simulink model "WindTurbineNM80"  (R2025b)
settings: Solver=VariableStepAuto  StartTime=0.0  StopTime=1000.0  MaxStep=0.02  RelTol=1e-3  AbsTol=1e-3  EnableMultiTasking=on
InitFcn:
  | WindTurbineNM80_init
values from neighbouring files (symbols this model uses):
  Ki = 0.5    [WindTurbineNM80_init.m]
  Kp = -[1.50 1.10 0.95 0.75 0.60 0.40 0.30 0.25]    [WindTurbineNM80_init.m]
  Lomg = 0:0.1:2*omgn    [WindTurbineNM80_init.m]
  Ltorque = zeros(1, length(Lomg))    [WindTurbineNM80_init.m]
  P0 = block.DialogPrm(1).Data    [Sbem.m]    (also in V10_init.mat = [0.0256690203 0 0.1920105638 0 1.7253273454 0.0016163595 0 0; V12_init.mat = [0.0307356949 0 0.2300256376 0 1.7632116641 0.0024078403 0 0; V15_init.mat = [0.0285896181 0 0.2236008103 0 1.8055130146 0.0031083935 0 5; V20_init.mat = [0.0174352214 0 0.1599644548 0 1.8055130193 0.0031083935 0 1)
  P1 = [rho, kp]    [NM80.m]    (also in NM92.m; Sbem.m = block.DialogPrm(2).Data)
  P2 = [R Nb Jb kb mt dt kt nu Jr dr kr Jg Un Pn omgn If p]    [NM80.m]    (also in NM92.m; Sbem.m = block.DialogPrm(3).Data)
  P3 = [r; c; thetat; th]    [NM80.m]    (also in NM92.m = [r; c; thetat]; Sbem.m = block.DialogPrm(4).Data)
  P4 = [Vn, lambdan, thetan]    [NM80.m]    (also in NM92.m)
  Pc = [omgA omgB omgC omgD omgE MB MC ME Kopt]    [WindTurbineNM80_init.m]
  Ptheta = [0 1 2 5 10 15 20 30]    [WindTurbineNM80_init.m]
  theta0 = 0.1    [V10_init.mat]    (also in V12_init.mat; V15_init.mat = 5.6378340943; V20_init.mat = 15.771114223; V25_init.mat = 22.7706169843)
  V0 = 10    [V10_init.mat]    (also in V12_init.mat = 12; V15_init.mat = 15; V20_init.mat = 20; V25_init.mat = 25)
libraries: sim3dlib x2, simulink x1
settings Model: Creator=ihoutzager  LastModifiedBy=ihout
settings SolverCC: AutoScaleAbsTol=off  AlgebraicLoopSolver=TrustRegion
settings DataIOCC: LimitDataPoints=on  SaveFormat=Array  SignalLoggingSaveFormat=ModelDataLogs  SaveOutput=off  SignalLogging=off  SaveTime=off  ReturnWorkspaceOutputs=off  SignalLoggingName=sigsOut
settings OptimizationCC: InitFltsAndDblsToZero=on  LifeSpan=inf
settings DebuggingCC: AlgebraicLoopMsg=none  SaveWithParameterizedLinksMsg=none  UnderspecifiedInitializationDetection=Classic  MergeDetectMultiDrivingBlocksExec=none  SignalResolutionControl=TryResolveAllWithWarning  MultiTaskDSMMsg=warning  MultiTaskCondExecSysMsg=none  FcnCallInpInsideContextMsg=warning  UnconnectedInputMsg=warning  UnconnectedOutputMsg=warning  UnconnectedLineMsg=warning  SFUnexpectedBacktrackingDiag=warning  SFNoUnconditionalDefaultTransitionDiag=warning  SFExecutionAtInitializationDiag=none  ArithmeticOperatorsInVariantConditions=warning
settings HardwareCC: ProdBitPerPointer=32.0  ProdBitPerSizeT=32.0  ProdBitPerPtrDiffT=32.0  ProdLargestAtomicFloat=None  ProdIntDivRoundTo=Undefined  ProdEndianess=Unspecified  ProdWordSize=32.0  ProdHWDeviceType=32-bit Generic  TargetUnknown=on
settings ModelReferenceCC: PropagateSignalLabelsOutOfModel=off
settings SFSimCC: SimParseCustomCode=off
settings RTWCC: GPUComputeCapability=3.5
settings CodeAppCC: StateflowObjectComments=on
settings GRTTargetCC: TargetFcnLib=ansi_tfl_tmw.mat  TargetLangStandard=C89/C90 (ANSI)  CombineOutputUpdateFcns=off  GRTInterface=on
settings ConfigComp: CovMetricSettings=dw  CovSaveCumulativeToWorkspaceVar=on  CovSaveSingleToWorkspaceVar=on

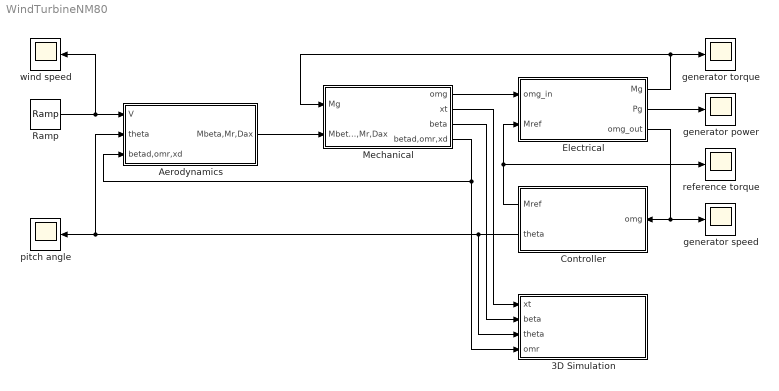
== system WindTurbineNM80 ==
  3D Simulation : Subsystem
  Aerodynamics : Subsystem
  Controller : Subsystem
  Electrical : Subsystem
  Mechanical : Subsystem
  Ramp : simulink/Sources/Ramp  slope=0.02  start=100  InitialOutput=V0
  generator power : Scope
      settings: TimeSpan=29.23076923076923  ActiveDisplayYMinimum=1.8990232335376493E+6  ActiveDisplayYMaximum=8.8179371513424478E+6  DataLoggingVariableName=ScopeData3
  generator speed : Scope
      settings: ActiveDisplayYMinimum=62.485741146490142  ActiveDisplayYMaximum=70.982692485822966  DataLoggingVariableName=ScopeData4
  generator torque : Scope
      settings: ActiveDisplayYMinimum=-2749.5211903948921  ActiveDisplayYMaximum=24745.690713554031
  pitch angle : Scope
      settings: ActiveDisplayYMinimum=16.304990778596967  ActiveDisplayYMaximum=20.832866708682104  DataLoggingVariableName=ScopeData2
  reference torque : Scope
      settings: ActiveDisplayYMinimum=2000  ActiveDisplayYMaximum=13000  DataLoggingVariableName=ScopeData5
  wind speed : Scope
      settings: ActiveDisplayYMinimum=3.5895500000000005  ActiveDisplayYMaximum=17.69405
  wires:
  Electrical/1(Mg) -> Mechanical/1(Mg), generator torque/1
  Mechanical/1(omg) -> Electrical/1(omg_in)
  Mechanical/4(betad,omr,xd) -> Aerodynamics/3(betad,omr,xd), 3D Simulation/4(omr)
  Controller/1(Mref) -> reference torque/1, Electrical/2(Mref)
  Electrical/3(omg_out) -> Controller/1(omg), generator speed/1
  Controller/2(theta) -> pitch angle/1, Aerodynamics/2(theta), 3D Simulation/3(theta)
  Aerodynamics/1(Mbeta,Mr,Dax) -> Mechanical/2(Mbeta,Mr,Dax)
  Ramp/1 -> wind speed/1, Aerodynamics/1(V)
  Electrical/2(Pg) -> generator power/1
  Mechanical/2(xt) -> 3D Simulation/1(xt)
  Mechanical/3(beta) -> 3D Simulation/2(beta)

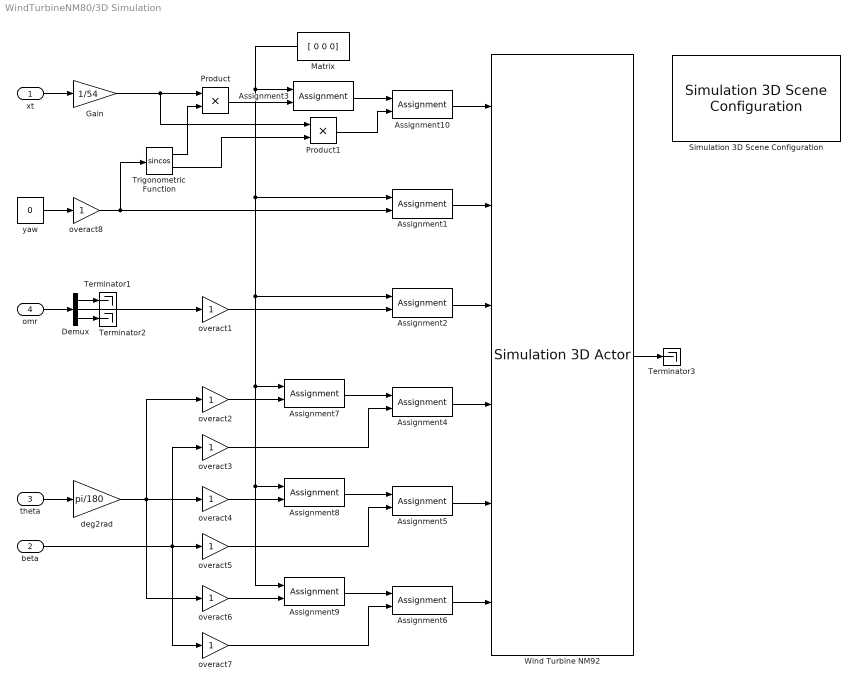
== system WindTurbineNM80/3D Simulation ==
  xt : Inport
  beta : Inport  Port=2
  theta : Inport  Port=3
  omr : Inport  Port=4
  Assignment{1,7..9} (4 alike) : Assignment  DiagnosticForDimensions=Warning  IndexOptions=Index vector (dialog)  Indices=3  OutputSizes=1
  Assignment10 : Assignment  DiagnosticForDimensions=Warning  IndexOptions=Index vector (dialog)  Indices=2  OutputSizes=1
  Assignment2 : Assignment  DiagnosticForDimensions=Warning  IndexOptions=Index vector (dialog)  Indices=2  OutputSizes=1
  Assignment{3..6} (4 alike) : Assignment  DiagnosticForDimensions=Warning  IndexOptions=Index vector (dialog)  Indices=1  OutputSizes=1
  Demux : Demux  Outputs=3
  Gain : Gain  Gain=1/54
  Matrix : Constant  Value=[ 0 0 0]  VectorParams1D=off
  Product : Product
  Product1 : Product
  Simulation 3D Scene Configuration : sim3dlib/Simulation 3D Scene Configuration  Priority=0  ProjectFormat=Default Scenes  SceneDesc=Empty scene  ProjectName=C:\Program Files\MATLAB\R2025b\toolbox\shared\sim3d_projects\automotive_project_windows\UE\WindowsNoEditor\VehicleSimulation.exe  ScenePath=/Game/Maps/HwStrght  EnableOpenDRIVE=off  vehTagList={'Custom';'Front';'Quadcopter';'Scene Origin';'WindTurbineNM92'}  vehTag=Front  AttachedCameraRelativeTranslation=[0 0 0]  FreeCameraDefaultInitialTranslation=[-6, 0, 2]  AttachedCameraRelativeRotation=[0 0 0]  FreeCameraDefaultInitialRotation=[0, -15, 0]  ViewpointName=Front  FreeCameraInitialTranslation=[0 120 60]  ViewpointTranslation=[0 0 0]  FreeCameraInitialRotation=[0 0 -90]  ViewpointRotation=[0 0 0]  OpVisEn=off  Ts=.02  EnableWindow=on  EnableRemoteAccess=off  EnableWeather=off  SunAzimuth=90  SunAltitude=40.0  EnableGeospatialSun=off  Latitude=0  Longitude=0  Date=2023-01-01  Time=10:30:00  GeoTimeZone=-5.0  SunDaylightSaving=off  wind=1  clouds=10  EnableVolumetricClouds=off  CloudCoverage=0  CloudAltitude=6  fog=0  rain=0  RaindropsEffect=off  SnowDensity=0  EnableGeospatial=off  TilesetSource=Earth terrain  UseTrueOrigin=off  OriginHeight=200  OriginLatitude=40.744652  OriginLongitude=-73.988864  MapStyle=Aerial  AdditionalAssetIDs=[]  UseAdvancedSunSky=off  SolarTime=11  TimeZone=-5  Day=21  Month=9  Year=2022  UseDaylightSavingTime=on  DSTStartDay=10  DSTStartMonth=3  DSTEndDay=3  DSTEndMonth=11  DSTSwitchHour=2  sensorTag=MainCamera1  sensorId=1  sensorName=MainCamera1  mountLoc=Origin  offsetFlag=off  tmountOffset=[0, 0, 0]  rmountOffset=[0, 0, 0]  HorizontalResolution=1280  VerticalResolution=720  HorizontalFOV=60  mountPoint=[0 0 0]  mountOrientation=[0 0 0]  aMode=5  ID=1  GeoTrigger=Inactive  ViewNameList={'Custom', 'Front'}  ViewTranslationList={'[0 0 0]', '[0 120 60]'}  ViewRotationList={'[0 0 0]', '[0 0 -90]'}
      settings: LibrarySourceBlock=sl3dlib/Simulation 3D/Simulation 3D Scene Configuration
  Terminator1 : Terminator
  Terminator2 : Terminator
  Terminator3 : Terminator
  Trigonometric Function : Trigonometry  Operator=sincos
  Wind Turbine NM92 : sim3dlib/Simulation 3D Actor  Priority=1  ActorName=WindTurbineNM92  ParentName=Front  Operation=Create at setup  InitScriptText=|  SampleTime=-1  Translation=[0 0 0]  Rotation=[0 0 0]  Scale=[1 1 1]  InputsText=|  aMode=5  ActorTag=WindTurbineNM92  ActorType=Sim3dActor  ID=C
      InitScriptText=|
      | NM92.FoundationPile = sim3d.Actor(ActorName='FoundationPile',...
      |     Translation=[0 0 0],...
      |     Mobility=sim3d.utils.MobilityTypes.Static);
      | add(World,NM92.FoundationPile,Actor);
      | load(NM92.FoundationPile,'actors3d\NM92_FoundationPile.x3d')
      | 
      | NM92.DeckSupportPlate1 = sim3d.Actor(ActorName='DeckSupportPlate1',...
      |     Mobility=sim3d.utils.MobilityTypes.Static);
      | add(World,NM92.DeckSupportPlate1,Actor);
      | load(NM92.DeckSupportPlate1,'actors3d\NM92_DeckSupportPlate1.x3d')
      | 
      | NM92.DeckSupportPlate2 = sim3d.Actor(ActorName='DeckSupportPlate2',...
      |     Mobility=sim3d.utils.MobilityTypes.Static);
      | add(World,NM92.DeckSupportPlate2,Actor);
      | load(NM92.DeckSupportPlate2,'actors3d\NM92_DeckSupportPlate2.x3d')
      | 
      | NM92.DeckSupport1 = sim3d.Actor(ActorName='DeckSupport1',...
      |     Mobility=sim3d.utils.MobilityTypes.Static);
      | add(World,NM92.DeckSupport1,Actor);
      | load(NM92.DeckSupport1,'actors3d\NM92_DeckSupport1.x3d')
      | 
      | NM92.DeckSupport2 = sim3d.Actor(ActorName='DeckSupport2',...
      |     Mobility=sim3d.utils.MobilityTypes.Static);
      | add(World,NM92.DeckSupport2,Actor);
      | load(NM92.DeckSupport2,'actors3d\NM92_DeckSupport2.x3d')
      | 
      | NM92.Deck = sim3d.Actor(ActorName='Deck',...
      |     Mobility=sim3d.utils.MobilityTypes.Static);
      | add(World,NM92.Deck,Actor);
      | load(NM92.Deck,'actors3d\NM92_Deck.x3d')
      | 
      | NM92.DeckRailing = sim3d.Actor(ActorName='DeckRailing',...
      |     Mobility=sim3d.utils.MobilityTypes.Static);
      | add(World,NM92.DeckRailing,Actor);
      | load(NM92.DeckRailing,'actors3d\NM92_DeckRailing.x3d')
      | 
      | NM92.ForeAftJoint = sim3d.Actor(ActorName='ForeAftJoint',...
      |     Translation=[0 0 14],...
      |     Mobility=sim3d.utils.MobilityTypes.Movable);
      | add(World,NM92.ForeAftJoint,NM92.FoundationPile)
      | 
      | NM92.Tower = sim3d.Actor(ActorName='Tower',...
      |     Translation=[0 0 -14],...
      |     Mobility=sim3d.utils.MobilityTypes.Movable);
      | add(World,NM92.Tower,NM92.ForeAftJoint);
      | load(NM92.Tower,'actors3d\NM92_Tower.x3d')
      | 
      | NM92.Door = sim3d.Actor(ActorName='Door',...
      |     Translation=[0 0 -14],...
      |     Mobility=sim3d.utils.MobilityTypes.Movable);
      | add(World,NM92.Door,NM92.ForeAftJoint);
      | load(NM92.Door,'actors3d\NM92_Door.x3d')
      | 
      | NM92.YawJoint = sim3d.Actor(ActorName='YawJoint',...
      |     Translation=[0 0 68],...
      |     Mobility=sim3d.utils.MobilityTypes.Movable);
      | add(World,NM92.YawJoint,NM92.Tower)
      | 
      | NM92.NacelleSpoiler = sim3d.Actor(ActorName='NacelleSpoiler',...
      |     Translation=[0 0 -68],...
      |     Mobility=sim3d.utils.MobilityTypes.Movable);
      | add(World,NM92.NacelleSpoiler,NM92.YawJoint);
      | load(NM92.NacelleSpoiler,'actors3d\NM92_NacelleSpoiler.x3d')
      | 
      | NM92.NacelleSpoilerMesh = sim3d.Actor(ActorName='NacelleSpoilerMesh',...
      |     Mobility=sim3d.utils.MobilityTypes.Movable);
      | add(World,NM92.NacelleSpoilerMesh,NM92.NacelleSpoiler);
      | load(NM92.NacelleSpoilerMesh,'actors3d\NM92_NacelleSpoilerMesh.x3d')
      | 
      | NM92.NacelleSides = sim3d.Actor(ActorName='NacelleSides',...
      |     Mobility=sim3d.utils.MobilityTypes.Movable);
      | add(world,NM92.NacelleSides,NM92.NacelleSpoiler);
      | load(NM92.NacelleSides,'actors3d\NM92_NacelleSides.x3d')
      | 
      | NM92.HubConnect = sim3d.Actor(ActorName='HubConnect',...
      |     Mobility=sim3d.utils.MobilityTypes.Movable);
      | add(World,NM92.HubConnect,NM92.NacelleSpoiler);
      | load(NM92.HubConnect,'actors3d\NM92_HubConnect.x3d')
      | 
      | NM92.RotationAxis = sim3d.Actor(ActorName='RotationAxis',...
      |     Translation=[-0.039169 2.146902 69.95571],...
      |     Rotation=[-0.0698124 0 0],...
      |     Mobility=sim3d.utils.MobilityTypes.Movable);
      | add(World,NM92.RotationAxis,NM92.HubConnect)
      | 
      | NM92.RotationJoint = sim3d.Actor(ActorName='RotationJoint',...
      |     Mobility=sim3d.utils.MobilityTypes.Movable);
      | add(World,NM92.RotationJoint,NM92.RotationAxis)
      | 
      | NM92.RotationInverse = sim3d.Actor(ActorName='RotationInverse',...
      |     Rotation=[0.0698124 0 0],...
      |     Mobility=sim3d.utils.MobilityTypes.Movable);
      | add(World,NM92.RotationInverse,NM92.RotationJoint)
      | 
      | NM92.Hub = sim3d.Actor(ActorName='Hub',...
      |     Translation=[0.039169 -2.146902 -69.95571],...
      |     Mobility=sim3d.utils.MobilityTypes.Movable);
      | add(World,NM92.Hub,NM92.RotationInverse);
      | load(NM92.Hub,'actors3d\NM92_Hub.x3d')
      |  
      | NM92.HubHatch1 = sim3d.Actor(ActorName='HubHatch1',...
      |     Mobility=sim3d.utils.MobilityTypes.Movable);
      | add(World,NM92.HubHatch1,NM92.Hub);
      | load(NM92.HubHatch1,'actors3d\NM92_HubHatch1.x3d')
      | 
      | NM92.HubHatch2 = sim3d.Actor(ActorName='HubHatch2',...
      |     Mobility=sim3d.utils.MobilityTypes.Movable);
      | add(World,NM92.HubHatch2,NM92.Hub);
      | load(NM92.HubHatch2,'actors3d\NM92_HubHatch2.x3d')
      | 
      | NM92.HubHatch3 = sim3d.Actor(ActorName='HubHatch3',...
      |     Mobility=sim3d.utils.MobilityTypes.Movable);
      | add(World,NM92.HubHatch3,NM92.Hub);
      | load(NM92.HubHatch3,'actors3d\NM92_HubHatch3.x3d')
      | 
      | NM92.RotorAxis = sim3d.Actor(ActorName='RotorAxis',...
      |     Translation=[-0.035752 3.576152 70.059258],...
      |     Rotation=[-0.0698124 0 0],...
      |     Mobility=sim3d.utils.MobilityTypes.Movable);
      | add(World,NM92.RotorAxis,NM92.Hub)
      | 
      | NM92.BladeAxis1= sim3d.Actor(ActorName='BladeAxis1',...
      |     Rotation=[0 -pi*2/3 0],...
      |     Mobility=sim3d.utils.MobilityTypes.Movable);
      | add(World,NM92.BladeAxis1,NM92.RotorAxis)
      | 
      | NM92.BladeJoint1= sim3d.Actor(ActorName='BladeJoint1',...
      |     Mobility=sim3d.utils.MobilityTypes.Movable);
      | add(World,NM92.BladeJoint1,NM92.BladeAxis1)
      | 
      | NM92.BladeInverse1 = sim3d.Actor(ActorName='BladeInverse1',...
      |     Rotation=[0.0698124 pi*2/3 pi],...
      |     Mobility=sim3d.utils.MobilityTypes.Movable);
      | add(World,NM92.BladeInverse1,NM92.BladeJoint1)
      | 
      | NM92.Blade1 = sim3d.Actor(ActorName='Blade1',...
      |     Translation=[0.035752 -3.576152 -70.059258],...
      |     Mobility=sim3d.utils.MobilityTypes.Movable);
      | add(World,NM92.Blade1,NM92.BladeInverse1);
      | load(NM92.Blade1,'actors3d\NM92_Blade1.x3d')
      | 
      | NM92.BladeAxis2= sim3d.Actor(ActorName='BladeAxis2',...
      |     Rotation=[0 pi*2/3 0],...
      |     Mobility=sim3d.utils.MobilityTypes.Movable);
      | add(World,NM92.BladeAxis2,NM92.RotorAxis)
      | 
      | NM92.BladeJoint2= sim3d.Actor(ActorName='BladeJoint2',...
      |     Mobility=sim3d.utils.MobilityTypes.Movable);
      | add(World,NM92.BladeJoint2,NM92.BladeAxis2)
      | 
      | NM92.BladeInverse2 = sim3d.Actor(ActorName='BladeInverse2',...
      |     Rotation=[0.0698124 -pi*2/3 pi],...
      |     Mobility=sim3d.utils.MobilityTypes.Movable);
      | add(World,NM92.BladeInverse2,NM92.BladeJoint2)
      | 
      | NM92.Blade2 = sim3d.Actor(ActorName='Blade2',...
      |     Translation=[0.035752 -3.576152 -70.059258],...
      |     Mobility=sim3d.utils.MobilityTypes.Movable);
      | add(World,NM92.Blade2,NM92.BladeInverse2);
      | load(NM92.Blade2,'actors3d\NM92_Blade2.x3d')
      | 
      | NM92.BladeAxis3= sim3d.Actor(ActorName='BladeAxis3',...
      |     Rotation=[0 0 0],...
      |     Mobility=sim3d.utils.MobilityTypes.Movable);
      | add(World,NM92.BladeAxis3,NM92.RotorAxis)
      | 
      | NM92.BladeJoint3= sim3d.Actor(ActorName='BladeJoint3',...
      |     Mobility=sim3d.utils.MobilityTypes.Movable);
      | add(World,NM92.BladeJoint3,NM92.BladeAxis3)
      | 
      | NM92.BladeInverse3 = sim3d.Actor(ActorName='BladeInverse3',...
      |     Rotation=[0.0698124 0 pi],...
      |     Mobility=sim3d.utils.MobilityTypes.Movable);
      | add(World,NM92.BladeInverse3,NM92.BladeJoint3)
      | 
      | NM92.Blade3 = sim3d.Actor(ActorName='Blade3',...
      |     Translation=[0.035752 -3.576152 -70.059258],...
      |     Mobility=sim3d.utils.MobilityTypes.Movable);
      | add(World,NM92.Blade3,NM92.BladeInverse3);
      | load(NM92.Blade3,'actors3d\NM92_Blade3.x3d')
      InputsText=|
      | ForeAftJoint.Rotation        
      | YawJoint.Rotation           
      | RotationJoint.AngularVelocity
      | BladeJoint1.Rotation         
      | BladeJoint2.Rotation         
      | BladeJoint3.Rotation
  deg2rad : Gain  Gain=pi/180
  overact{1..8} (8 alike) : Gain
  yaw : Constant  Value=0
  wires:
  Gain/1 -> Product/1, Product1/1
  Demux/2 -> overact1/1
  omr/1 -> Demux/1
  deg2rad/1 -> overact6/1, overact2/1, overact4/1
  Demux/1 -> Terminator1/1
  Demux/3 -> Terminator2/1
  Wind Turbine NM92/1 -> Terminator3/1
  Matrix/1 -> Assignment1/1, Assignment2/1, Assignment9/1, Assignment8/1, Assignment7/1, Assignment3/1
  Assignment1/1 -> Wind Turbine NM92/2
  yaw/1 -> overact8/1
  overact8/1 -> Trigonometric Function/1, Assignment1/2
  overact1/1 -> Assignment2/2
  Assignment7/1 -> Assignment4/1
  Assignment8/1 -> Assignment5/1
  Assignment9/1 -> Assignment6/1
  overact3/1 -> Assignment4/2
  overact2/1 -> Assignment7/2
  overact5/1 -> Assignment5/2
  overact7/1 -> Assignment6/2
  overact4/1 -> Assignment8/2
  overact6/1 -> Assignment9/2
  xt/1 -> Gain/1
  Assignment2/1 -> Wind Turbine NM92/3
  Assignment4/1 -> Wind Turbine NM92/4
  Assignment5/1 -> Wind Turbine NM92/5
  Assignment6/1 -> Wind Turbine NM92/6
  Assignment10/1 -> Wind Turbine NM92/1
  Assignment3/1 -> Assignment10/1
  Product/1 -> Assignment3/2
  Trigonometric Function/2 -> Product1/2
  Trigonometric Function/1 -> Product/2
  Product1/1 -> Assignment10/2
  beta/1 -> overact7/1, overact3/1, overact5/1
  theta/1 -> deg2rad/1

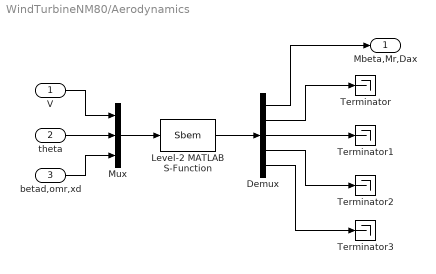
== system WindTurbineNM80/Aerodynamics ==
  V : Inport
  theta : Inport  Port=2
  betad,omr,xd : Inport  Port=3
  Demux : Demux  Outputs=[3,1,1,1,1]
      settings: DisplayOption=none
  Level-2 MATLAB S-Function : M-S-Function  FunctionName=Sbem  Parameters=P0,P1,P2,P3,P4
  Mux : Mux  Inputs=3
  Terminator{,1..3} (4 alike) : Terminator
  Mbeta,Mr,Dax : Outport
  wires:
  theta/1 -> Mux/2
  V/1 -> Mux/1
  betad,omr,xd/1 -> Mux/3
  Mux/1 -> Level-2 MATLAB S-Function/1
  Level-2 MATLAB S-Function/1 -> Demux/1
  Demux/1 -> Mbeta,Mr,Dax/1
  Demux/3 -> Terminator1/1
  Demux/4 -> Terminator2/1
  Demux/5 -> Terminator3/1
  Demux/2 -> Terminator/1

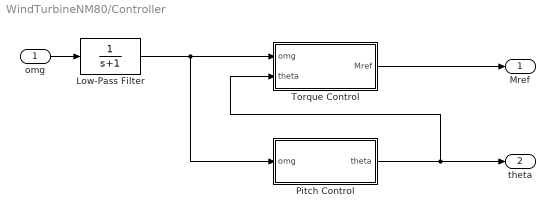
== system WindTurbineNM80/Controller ==
  omg : Inport
  Low-Pass Filter : TransferFcn  Denominator=[1 1]
  Pitch Control : Subsystem
  Torque Control : Subsystem
  Mref : Outport
  theta : Outport  Port=2
  wires:
  omg/1 -> Low-Pass Filter/1
  Low-Pass Filter/1 -> Pitch Control/1(omg), Torque Control/1(omg)
  Pitch Control/1(theta) -> Torque Control/2(theta), theta/1
  Torque Control/1(Mref) -> Mref/1

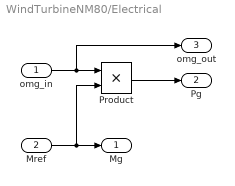
== system WindTurbineNM80/Electrical ==
  omg_in : Inport
  Mref : Inport  Port=2
  Product : Product  RndMeth=Zero
  Mg : Outport
  Pg : Outport  Port=2
  omg_out : Outport  Port=3
  wires:
  Product/1 -> Pg/1
  omg_in/1 -> Product/1, omg_out/1
  Mref/1 -> Mg/1, Product/2

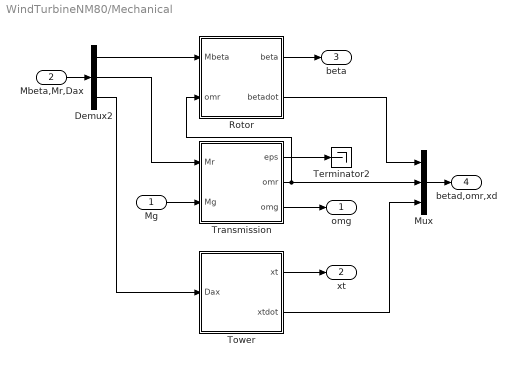
== system WindTurbineNM80/Mechanical ==
  Mg : Inport
  Mbeta,Mr,Dax : Inport  Port=2
  Demux2 : Demux  Outputs=3
      settings: DisplayOption=none
  Mux : Mux  Inputs=3
  Rotor : Subsystem
  Terminator2 : Terminator
  Tower : Subsystem
  Transmission : Subsystem
  omg : Outport
  xt : Outport  Port=2
  beta : Outport  Port=3
  betad,omr,xd : Outport  Port=4
  wires:
  Transmission/3(omg) -> omg/1
  Rotor/2(betadot) -> Mux/1
  Transmission/2(omr) -> Mux/2, Rotor/2(omr)
  Mux/1 -> betad,omr,xd/1
  Transmission/1(eps) -> Terminator2/1
  Tower/2(xtdot) -> Mux/3
  Tower/1(xt) -> xt/1
  Mbeta,Mr,Dax/1 -> Demux2/1
  Mg/1 -> Transmission/2(Mg)
  Demux2/1 -> Rotor/1(Mbeta)
  Demux2/3 -> Tower/1(Dax)
  Demux2/2 -> Transmission/1(Mr)
  Rotor/1(beta) -> beta/1

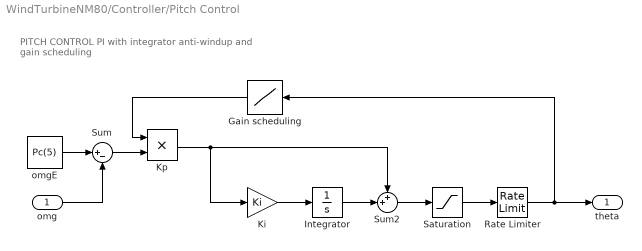
== system WindTurbineNM80/Controller/Pitch Control ==
  note: PITCH CONTROL
      | PI with integrator anti-windup and gain scheduling
  omg : Inport
  Gain scheduling : Lookup  InputValues=Ptheta  Table=Kp  LookUpMeth=Interpolation-Use End Values  SaturateOnIntegerOverflow=off
  Integrator : Integrator  InitialCondition=theta0  LimitOutput=on  UpperSaturationLimit=90  LowerSaturationLimit=P4(3)
  Ki : Gain  Gain=Ki
  Kp : Product  RndMeth=Zero
  Rate Limiter : RateLimiter  RisingSlewLimit=4  FallingSlewLimit=-4  SampleTimeMode=inherited
  Saturation : Saturate  UpperLimit=90  LowerLimit=P4(3)
  Sum : Sum  Inputs=|+-
  Sum2 : Sum  Inputs=++|
  omgE : Constant  Value=Pc(5)
  theta : Outport
  wires:
  omgE/1 -> Sum/1
  Sum/1 -> Kp/2
  Integrator/1 -> Sum2/2
  Sum2/1 -> Saturation/1
  Ki/1 -> Integrator/1
  Kp/1 -> Sum2/1, Ki/1
  omg/1 -> Sum/2
  Gain scheduling/1 -> Kp/1
  Saturation/1 -> Rate Limiter/1
  Rate Limiter/1 -> Gain scheduling/1, theta/1

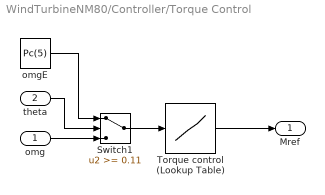
== system WindTurbineNM80/Controller/Torque Control ==
  omg : Inport
  theta : Inport  Port=2
  Switch1 : Switch  Threshold=0.11  SaturateOnIntegerOverflow=off  InputSameDT=off
  Torque control (Lookup Table) : Lookup  InputValues=Lomg  Table=Ltorque  LookUpMeth=Interpolation-Use End Values  SaturateOnIntegerOverflow=off
  omgE : Constant  Value=Pc(5)
  Mref : Outport
  wires:
  Torque control (Lookup Table)/1 -> Mref/1
  theta/1 -> Switch1/2
  omgE/1 -> Switch1/1
  omg/1 -> Switch1/3
  Switch1/1 -> Torque control (Lookup Table)/1

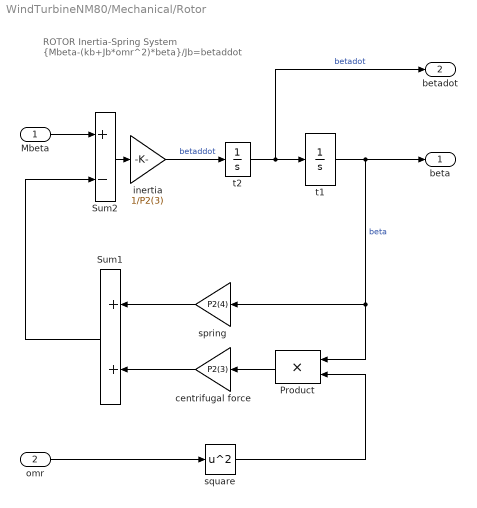
== system WindTurbineNM80/Mechanical/Rotor ==
  note: ROTOR
      | Inertia-Spring System
      | {Mbeta-(kb+Jb*omr^2)*beta}/Jb=betaddot
  Mbeta : Inport
  omr : Inport  Port=2
  Product : Product  SaturateOnIntegerOverflow=on  OutDataTypeStr=Inherit: Same as first input
  Sum1 : Sum  InputSameDT=on  SaturateOnIntegerOverflow=on  OutDataTypeStr=Inherit: Same as first input
  Sum2 : Sum  Inputs=+-  InputSameDT=on  SaturateOnIntegerOverflow=on  OutDataTypeStr=Inherit: Same as first input
  centrifugal force : Gain  Gain=P2(3)  SaturateOnIntegerOverflow=on  OutDataTypeStr=Inherit: Same as input  ParamDataTypeStr=Inherit: Same as input
  inertia : Gain  Gain=1/P2(3)  SaturateOnIntegerOverflow=on  OutDataTypeStr=Inherit: Same as input  ParamDataTypeStr=Inherit: Same as input
  spring : Gain  Gain=P2(4)  SaturateOnIntegerOverflow=on  OutDataTypeStr=Inherit: Same as input  ParamDataTypeStr=Inherit: Same as input
  square : Math  Operator=square  SignedPower=on
  t1 : Integrator  InitialCondition=P0(1)  ZeroCross=off
  t2 : Integrator  InitialCondition=P0(2)
  beta : Outport
  betadot : Outport  Port=2
  wires:
  square/1 -> Product/2
  Product/1 -> centrifugal force/1
  omr/1 -> square/1
  centrifugal force/1 -> Sum1/2
  Sum1/1 -> Sum2/2
  spring/1 -> Sum1/1
  Sum2/1 -> inertia/1
  inertia/1 -> t2/1  "betaddot"
  Mbeta/1 -> Sum2/1
  t1/1 -> Product/1, spring/1, beta/1  "beta"
  t2/1 -> betadot/1, t1/1  "betadot"

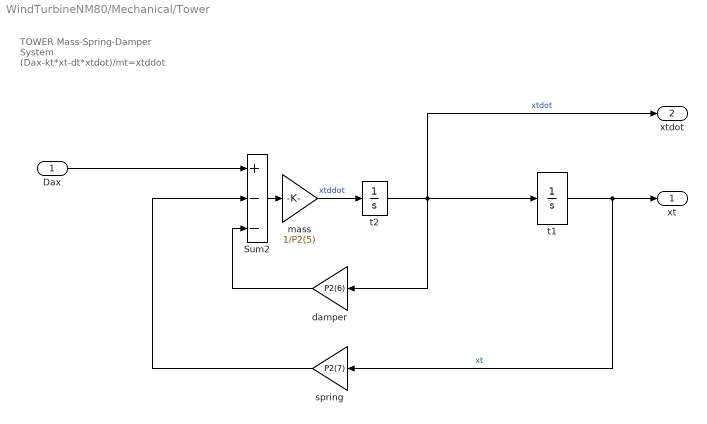
== system WindTurbineNM80/Mechanical/Tower ==
  note: TOWER
      | Mass-Spring-Damper System
      | (Dax-kt*xt-dt*xtdot)/mt=xtddot
  Dax : Inport
  Sum2 : Sum  Inputs=+--  InputSameDT=on  SaturateOnIntegerOverflow=on  OutDataTypeStr=Inherit: Same as first input
  damper : Gain  Gain=P2(6)  SaturateOnIntegerOverflow=on  OutDataTypeStr=Inherit: Same as input  ParamDataTypeStr=Inherit: Same as input
  mass : Gain  Gain=1/P2(5)  SaturateOnIntegerOverflow=on  OutDataTypeStr=Inherit: Same as input  ParamDataTypeStr=Inherit: Same as input
  spring : Gain  Gain=P2(7)  SaturateOnIntegerOverflow=on  OutDataTypeStr=Inherit: Same as input  ParamDataTypeStr=Inherit: Same as input
  t1 : Integrator  InitialCondition=P0(3)  ZeroCross=off
  t2 : Integrator  InitialCondition=P0(4)
  xt : Outport
  xtdot : Outport  Port=2
  wires:
  spring/1 -> Sum2/2
  mass/1 -> t2/1  "xtddot"
  Sum2/1 -> mass/1
  Dax/1 -> Sum2/1
  t1/1 -> spring/1, xt/1  "xt"
  t2/1 -> xtdot/1, damper/1, t1/1  "xtdot"
  damper/1 -> Sum2/3

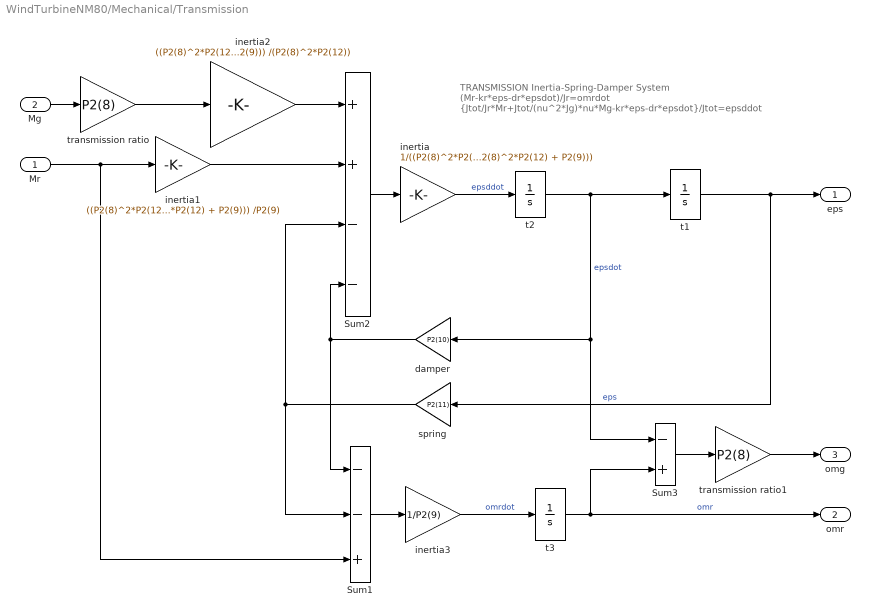
== system WindTurbineNM80/Mechanical/Transmission ==
  note: TRANSMISSION
      | Inertia-Spring-Damper System
      | (Mr-kr*eps-dr*epsdot)/Jr=omrdot
      | {Jtot/Jr*Mr+Jtot/(nu^2*Jg)*nu*Mg-kr*eps-dr*epsdot}/Jtot=epsddot
  Mr : Inport
  Mg : Inport  Port=2
  Sum1 : Sum  Inputs=--+  InputSameDT=on  SaturateOnIntegerOverflow=on  OutDataTypeStr=Inherit: Same as first input
  Sum2 : Sum  Inputs=++--  InputSameDT=on  SaturateOnIntegerOverflow=on  OutDataTypeStr=Inherit: Same as first input
  Sum3 : Sum  Inputs=-+  InputSameDT=on  SaturateOnIntegerOverflow=on  OutDataTypeStr=Inherit: Same as first input
  damper : Gain  Gain=P2(10)  SaturateOnIntegerOverflow=on  OutDataTypeStr=Inherit: Same as input  ParamDataTypeStr=Inherit: Same as input
  inertia : Gain  Gain=1/((P2(8)^2*P2(12)*P2(9))/(P2(8)^2*P2(12) + P2(9)))  SaturateOnIntegerOverflow=on  OutDataTypeStr=Inherit: Same as input  ParamDataTypeStr=Inherit: Same as input
  inertia1 : Gain  Gain=((P2(8)^2*P2(12)*P2(9))/(P2(8)^2*P2(12) + P2(9))) /P2(9)  SaturateOnIntegerOverflow=on  OutDataTypeStr=Inherit: Same as input  ParamDataTypeStr=Inherit: Same as input
  inertia2 : Gain  Gain=((P2(8)^2*P2(12)*P2(9))/(P2(8)^2*P2(12) + P2(9))) /(P2(8)^2*P2(12))  SaturateOnIntegerOverflow=on  OutDataTypeStr=Inherit: Same as input  ParamDataTypeStr=Inherit: Same as input
  inertia3 : Gain  Gain=1/P2(9)  SaturateOnIntegerOverflow=on  OutDataTypeStr=Inherit: Same as input  ParamDataTypeStr=Inherit: Same as input
  spring : Gain  Gain=P2(11)  SaturateOnIntegerOverflow=on  OutDataTypeStr=Inherit: Same as input  ParamDataTypeStr=Inherit: Same as input
  t1 : Integrator  InitialCondition=P0(6)  ZeroCross=off
  t2 : Integrator  InitialCondition=P0(7)  LowerSaturationLimit=0
  t3 : Integrator  InitialCondition=P0(5)  ZeroCross=off
  transmission ratio : Gain  Gain=P2(8)  SaturateOnIntegerOverflow=on  OutDataTypeStr=Inherit: Same as input  ParamDataTypeStr=Inherit: Same as input
  transmission ratio1 : Gain  Gain=P2(8)  SaturateOnIntegerOverflow=on  OutDataTypeStr=Inherit: Same as input  ParamDataTypeStr=Inherit: Same as input
  eps : Outport
  omr : Outport  Port=2
  omg : Outport  Port=3
  wires:
  transmission ratio1/1 -> omg/1
  Sum3/1 -> transmission ratio1/1
  t3/1 -> Sum3/2, omr/1  "omr"
  Sum1/1 -> inertia3/1
  inertia3/1 -> t3/1  "omrdot"
  inertia1/1 -> Sum2/2
  Mr/1 -> Sum1/3, inertia1/1
  Mg/1 -> transmission ratio/1
  transmission ratio/1 -> inertia2/1
  t2/1 -> Sum3/1, damper/1, t1/1  "epsdot"
  inertia2/1 -> Sum2/1
  spring/1 -> Sum1/2, Sum2/3
  inertia/1 -> t2/1  "epsddot"
  Sum2/1 -> inertia/1
  t1/1 -> spring/1, eps/1  "eps"
  damper/1 -> Sum1/1, Sum2/4
